simulink model "sm_DDPG_Training_Circuit_h0"  (R2022b)
settings: Solver=VariableStepAuto  StartTime=0.0  StopTime=2000  RelTol=1e-3
values from neighbouring files (symbols this model uses):
  areaFinEvap = 0.05    [pramInit.m]
  areaRoofRoom1 = roofArea/4    [pramInit.m]
  areaRoofRoom2 = roofArea/4    [pramInit.m]
  areaRoofRoom3 = roofArea/4    [pramInit.m]
  areaRoofRoom4 = roofArea/4    [pramInit.m]
  areaWallRoom1 = (lenHouse*3/5 *htHouse+widHouse*2/3*htHouse) - areaWindowRoom1    (= 95.6666666667)    [pramInit.m]
  areaWallRoom2 = (lenHouse*3/5*htHouse+widHouse/3*htHouse) - areaWindowRoom2    (= 83.3333333333)    [pramInit.m]
  areaWallRoom3 = (lenHouse*2/5*htHouse+widHouse*2/3*htHouse) - areaWindowRoom3    (= 72.6666666667)    [pramInit.m]
  areaWallRoom4 = (lenHouse*2/5*htHouse+widHouse/3*htHouse) - areaWindowRoom4    (= 59.3333333333)    [pramInit.m]
  areaWindowRoom1 = 3 * 1 *1    (= 3)    [pramInit.m]
  areaWindowRoom2 = 2 * 1 *1    (= 2)    [pramInit.m]
  areaWindowRoom3 = 2* 1 *1    (= 2)    [pramInit.m]
  areaWindowRoom4 = 2 * 1 *1    (= 2)    [pramInit.m]
  diaCond = 0.014    [pramInit.m]
  diaEvap = 0.126    [pramInit.m]
  diaGroundLoop = 0.032    [pramInit.m]
  diaOuterCond = 0.0158    [pramInit.m]
  diaOuterEvap = 0.1344    [pramInit.m]
  diaRadiatorPipe = 0.0125    [pramInit.m]
  htCondDuct = 0.3    [pramInit.m]
  htEvapDuct = 2.5    [pramInit.m]
  kTube = 400    [pramInit.m]
  leakRoofPercent = 0.1    [pramInit.m]
  leakWallPercent = 0.15    [pramInit.m]
  leakWinPercent = 0.2    [pramInit.m]
  numFinsEvap = 90    [pramInit.m]
  numTubeRowsCond = 20    [pramInit.m]
  numTubeRowsEvap = 400    [pramInit.m]
  numTubesPerRowCond = 10    [pramInit.m]
  numTubesPerRowEvap = 20    [pramInit.m]
  qGroundLoopPump = 18    [pramInit.m]
  roofDensity = 32    [pramInit.m]
  thkRoof = 0.2    [pramInit.m]
  thkWall = 0.2    [pramInit.m]
  thkWindow = 0.01    [pramInit.m]
  tInitHW = 50    [pramInit.m]
  tRoom = 23    [pramInit.m]
  Ts = 1.0    (= 1)    [code_DDPG_Training.m]    (also in code_Experimental_Setup.m)
  wallDensity = 1920    [pramInit.m]
  wCondDuct = 1.6    [pramInit.m]
  wEvapDuct = 0.96    [pramInit.m]
  windowDensity = 2700    [pramInit.m]
undefined symbols (not defined in the file or in its folder): DiscIntNeverNeededParam
libraries: fl_lib x144, nesl_utility x27, SimscapeFluids_lib x15, simulink x4, rllib x1
(part 2 of 4)

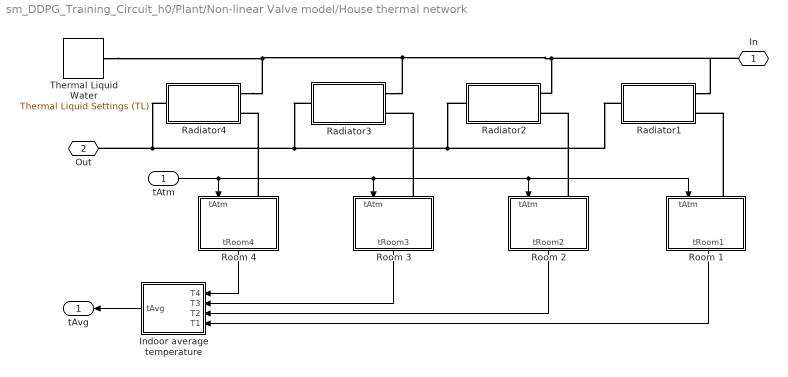
== system sm_DDPG_Training_Circuit_h0/Plant/Non-linear Valve model/House thermal network ==
  tAtm : Inport
  Indoor average temperature : Subsystem
  Radiator1 : Subsystem
      mask Display: disp('Radiator')
  Radiator2 : Subsystem
      mask Display: disp('Radiator')
  Radiator3 : Subsystem
      mask Display: disp('Radiator')
  Radiator4 : Subsystem
      mask Display: disp('Radiator')
  Room 1 : Subsystem  Tag=PublishSubsystem
      mask Display: disp('Room 1')
  Room 2 : Subsystem  Tag=PublishSubsystem
      mask Display: disp('Room 2')
  Room 3 : Subsystem  Tag=PublishSubsystem
      mask Display: disp('Room 3')
  Room 4 : Subsystem  Tag=PublishSubsystem
      mask Display: disp('Room 4')
  Thermal Liquid Water : fl_lib/Thermal Liquid/Utilities/Thermal Liquid Settings (TL)  table_dimensions=0  T_TLU=[273.1600 : 10 : 373.16]' K  p_TLU=[0.01, 0.1, 5 : 5 : 50] MPa  p_atm=0.101325 MPa  pT_region_flag=1  T_min=273.16 K  T_max=373.16 K  p_min=0.01 MPa  p_max=50 MPa  T_min_1D=273.16 K  T_max_1D=363.16 K  p_min_1D=0.05 MPa  p_max_1D=50 MPa  pT_validity_TLU=[1, 1, 1, 1, 1, 1, 1, 1, 1, 1, 1, 1; 1, 1, 1, 1, 1, 1, 1, 1, 1, 1, 1, 1; 1, 1, 1, 1, 1, 1, 1, 1, 1, 1, 1, 1; 1, 1, 1, 1, 1, 1, 1, 1, 1, 1, 1, 1; 1, 1, 1, 1, 1, 1, 1, 1, 1, 1, 1, 1; 0, 1, 1, 1, 1, 1, 1, 1, 1, 1, 1, 1; 0, 1, 1, 1, 1, 1, 1, 1, 1, 1, 1, 1; 0, 1, 1, 1, 1, 1, 1, 1, 1, 1, 1, 1; 0, 1, 1, 1, 1, 1, 1, 1, 1, 1, 1, 1; 0, 1, 1, 1, 1, 1, 1, 1, 1, 1, 1, 1; 0, 1, 1, 1, 1, 1, 1, 1, 1, 1, 1, 1]  rho_parameterization_2D=1  rho_parameterization_1D=1  rho_TLU=[999.8, 999.8, 1002.3, 1004.8, 1007.3, 1009.7, 1012.2, 1014.5, 1016.9, 1019.2, 1021.5, 1023.8; 999.7, 999.7, 1002.0, 1004.4, 1006.7, 1009.0, 1011.3, 1013.5, 1015.8, 1018.0, 1020.2, 1022.3; 998.2, 998.2, 1000.4, 1002.7, 1004.9, 1007.1, 1009.3, 1011.5, 1013.6, 1015.7, 1017.8, 1019.9; 995.6, 995.6, 997.8, 1000.0, 1002.2, 1004.3, 1006.5, 1008.6, 1010.7, 1012.7, 1014.8, 1016.8; 992.2, 992.2, 994.4, 996.5, 998.6, 1000.8, 1002.9, 1004.9, 1007.0, 1009.0, 1011.0, 1013.0; 988.0, 988.0, 990.2, 992.3, 994.4, 996.5, 998.6, 1000.7, 1002.7, 1004.7, 1006.7, 1008.7; 983.2, 983.2, 985.3, 987.5, 989.6, 991.7, 993.8, 995.8, 997.9, 999.9, 1001.9, 1003.9; 977.8, 977.8, 979.9, 982.1, 984.2, 986.3, 988.4, 990.5, 992.5, 994.6, 996.6, 998.6; 971.8, 971.8, 974.0, 976.2, 978.3, 980.5, 982.6, 984.7, 986.8, 988.8, 990.9, 992.9; 965.3, 965.3, 967.5, 969.8, 972.0, 974.2, 976.3, 978.5, 980.6, 982.7, 984.7, 986.8; 958.8, 958.8, 960.6, 962.9, 965.2, 967.4, 969.6, 971.8, 974.0, 976.1, 978.2, 980.3] kg/m^3  beta_TLU=[1.9649, 1.9654, 1.9929, 2.0213, 2.0499, 2.0787, 2.1078, 2.1372, 2.1668, 2.1966, 2.2268, 2.2572; 2.0913, 2.0918, 2.1191, 2.1471, 2.1752, 2.2036, 2.2322, 2.2610, 2.2899, 2.3191, 2.3485, 2.3781; 2.1786, 2.1791, 2.2067, 2.2350, 2.2634, 2.2919, 2.3206, 2.3494, 2.3784, 2.4075, 2.4367, 2.4661; 2.2332, 2.2337, 2.2619, 2.2908, 2.3197, 2.3487, 2.3778, 2.4070, 2.4363, 2.4657, 2.4951, 2.5246; 2.2600, 2.2605, 2.2895, 2.3191, 2.3487, 2.3784, 2.4081, 2.4378, 2.4675, 2.4973, 2.5272, 2.5571; 2.2638, 2.2638, 2.2936, 2.3240, 2.3544, 2.3848, 2.4151, 2.4455, 2.4758, 2.5062, 2.5365, 2.5669; 2.2472, 2.2472, 2.2779, 2.3092, 2.3403, 2.3715, 2.4025, 2.4336, 2.4646, 2.4955, 2.5264, 2.5573; 2.2140, 2.2140, 2.2455, 2.2776, 2.3096, 2.3415, 2.3733, 2.4050, 2.4367, 2.4683, 2.4998, 2.5313; 2.1668, 2.1668, 2.1992, 2.2321, 2.2649, 2.2976, 2.3301, 2.3626, 2.3949, 2.4272, 2.4593, 2.4914; 2.1081, 2.1081, 2.1413, 2.1750, 2.2086, 2.2421, 2.2754, 2.3085, 2.3415, 2.3744, 2.4072, 2.4399; 2.0494, 2.0494, 2.0739, 2.1084, 2.1428, 2.1770, 2.2110, 2.2449, 2.2786, 2.3121, 2.3455, 2.3788] GPa  alpha_TLU=(1e-4 * [- 0.6790, - 0.6760, - 0.4900, - 0.3070, - 0.1300, 0.0410, 0.2060, 0.3650, 0.5190, 0.6680, 0.8110, 0.9490; 0.8780, 0.8810, 0.9980, 1.1140, 1.2270, 1.3370, 1.4450, 1.5490, 1.6510, 1.7500, 1.8460, 1.9390; 2.0680, 2.0690, 2.1410, 2.2130, 2.2830, 2.3520, 2.4200, 2.4860, 2.5510, 2.6140, 2.6760, 2.7360; 3.0340, 3.0350, 3.0740, 3.1130, 3.1520, 3.1910, 3.2290, 3.2670, 3.3050, 3.3410, 3.3770, 3.4130; 3.8550, 3.8560, 3.8700, 3.8840, 3.8990, 3.9140, 3.9300, 3.9460, 3.9610, 3.9770, 3.9930, 4.0090; 4.5780, 4.5780, 4.5720, 4.5660, 4.5620, 4.5580, 4.5550, 4.5520, 4.5500, 4.5490, 4.5480, 4.5470; 5.2330, 5.2330, 5.2090, 5.1860, 5.1650, 5.1440, 5.1250, 5.1070, 5.0900, 5.0740, 5.0590, 5.0450; 5.8400, 5.8400, 5.8010, 5.7620, 5.7250, 5.6910, 5.6570, 5.6250, 5.5950, 5.5660, 5.5380, 5.5120; 6.4140, 6.4140, 6.3600, 6.3070, 6.2560, 6.2080, 6.1610, 6.1170, 6.0740, 6.0330, 5.9940, 5.9560; 6.9670, 6.9670, 6.8980, 6.8310, 6.7660, 6.7050, 6.6460, 6.5890, 6.5350, 6.4820, 6.4320, 6.3840; 7.5190, 7.5190, 7.4230, 7.3420, 7.2640, 7.1890, 7.1180, 7.0490, 6.9830, 6.9200, 6.8590, 6.8000]) 1/K  rho_TLU_2=[999.7973, 999.8431, 1002.3216, 1004.8218, 1007.293, 1009.7358, 1012.1506, 1014.5379, 1016.8979, 1019.2311, 1021.538, 1023.8188; 999.6579, 999.7009, 1002.0303, 1004.382, 1006.7084, 1009.0101, 1011.2874, 1013.5407, 1015.7703, 1017.9766, 1020.1599, 1022.3206; 998.1632, 998.2045, 1000.4375, 1002.6924, 1004.9239, 1007.1324, 1009.3183, 1011.4819, 1013.6236, 1015.7438, 1017.8428, 1019.921; 995.6057, 995.6458, 997.81864, 1000.0128, 1002.1841, 1004.3332, 1006.4603, 1008.566, 1010.6505, 1012.7144, 1014.758, 1016.7815; 992.1724, 992.2119, 994.35133, 996.5113, 998.6484, 1000.7633, 1002.8563, 1004.928, 1006.9788, 1009.009, 1011.0192, 1013.0097; 988.02, 988.0299, 990.15684, 992.3035, 994.4268, 996.5273, 998.6056, 1000.6622, 1002.6976, 1004.7123, 1006.7067, 1008.6813; 983.18, 983.1901, 985.3217, 987.4721, 989.5983, 991.7008, 993.7803, 995.8374, 997.8726, 999.8864, 1001.8795, 1003.8522; 977.75, 977.7583, 979.9094, 982.0783, 984.2216, 986.34, 988.4343, 990.505, 992.5529, 994.5786, 996.5825, 998.5654; 971.77, 971.7836, 973.96734, 976.1678, 978.3409, 980.4876, 982.6087, 984.7049, 986.7768, 988.8254, 990.8511, 992.8545; 965.26, 965.3023, 967.53107, 969.7753, 971.9901, 974.1764, 976.3354, 978.4676, 980.5741, 982.6556, 984.7129, 986.7465; 958.62, 958.6315, 960.627, 962.9267, 965.1944, 967.4314, 969.6387, 971.8173, 973.9681, 976.0921, 978.19, 980.2628] kg/m^3  rho_ref_3=998.21 kg/m^3  T_ref_3=293.16 K  p_ref_3=0.101325 MPa  beta_const_3=2.1791 GPa  alpha_const_3=2.0691e-4 1/K  rho_TLU_4=[999.84; 999.7; 998.2; 995.65; 992.21; 988.03; 983.19; 977.76; 971.78; 965.3; 958.8] kg/m^3  beta_const_4=2.1791 GPa  p_ref_4=0.101325 MPa  rho_ref_5=998.21 kg/m^3  T_ref_5=293.16 K  p_ref_5=0.101325 MPa  beta_const_5=2.1791 GPa  alpha_const_5=2.0691e-4 1/K  u_parameterization_2D=1  u_parameterization_1D=1  u_TLU=[0.0002, 0.0018, 0.0860, 0.1588, 0.2190, 0.2670, 0.3034, 0.3288, 0.3436, 0.3483, 0.3435, 0.3294; 42.0620, 42.0600, 41.9350, 41.8040, 41.6680, 41.5270, 41.3820, 41.2330, 41.0810, 40.9240, 40.7630, 40.5990; 83.9530, 83.9480, 83.6510, 83.3490, 83.0490, 82.7490, 82.4510, 82.1530, 81.8560, 81.5600, 81.2650, 80.9710; 125.7700, 125.7600, 125.3100, 124.8600, 124.4100, 123.9700, 123.5300, 123.1000, 122.6800, 122.2500, 121.8400, 121.4200; 167.5700, 167.5600, 166.9600, 166.3700, 165.7900, 165.2100, 164.6500, 164.0900, 163.5400, 163.0000, 162.4600, 161.9400; 209.3600, 209.3600, 208.6300, 207.9000, 207.1900, 206.4800, 205.7900, 205.1100, 204.4500, 203.7900, 203.1400, 202.5000; 251.1900, 251.1900, 250.3300, 249.4700, 248.6200, 247.7900, 246.9800, 246.1800, 245.3900, 244.6200, 243.8600, 243.1200; 293.0600, 293.0600, 292.0700, 291.0700, 290.1000, 289.1400, 288.2000, 287.2800, 286.3800, 285.4900, 284.6200, 283.7700; 334.9900, 334.9900, 333.8600, 332.7300, 331.6300, 330.5400, 329.4800, 328.4400, 327.4100, 326.4100, 325.4300, 324.4600; 377.0000, 377.0000, 375.7300, 374.4600, 373.2200, 372.0000, 370.8100, 369.6400, 368.5000, 367.3800, 366.2700, 365.1900; 419.0100, 419.0100, 417.6900, 416.2700, 414.8900, 413.5400, 412.2100, 410.9100, 409.6400, 408.4000, 407.1700, 405.9800] kJ/kg  cp_TLU=[4.2199, 4.2194, 4.1957, 4.1726, 4.1508, 4.1300, 4.1103, 4.0916, 4.0738, 4.0569, 4.0408, 4.0254; 4.1955, 4.1951, 4.1769, 4.1592, 4.1422, 4.1259, 4.1103, 4.0954, 4.0812, 4.0676, 4.0545, 4.0421; 4.1843, 4.1840, 4.1690, 4.1543, 4.1401, 4.1264, 4.1133, 4.1007, 4.0885, 4.0768, 4.0656, 4.0548; 4.1801, 4.1798, 4.1667, 4.1538, 4.1413, 4.1293, 4.1177, 4.1064, 4.0956, 4.0851, 4.0750, 4.0653; 4.1796, 4.1794, 4.1675, 4.1558, 4.1444, 4.1334, 4.1227, 4.1123, 4.1023, 4.0926, 4.0832, 4.0741; 4.1813, 4.1813, 4.1702, 4.1592, 4.1484, 4.1380, 4.1279, 4.1181, 4.1086, 4.0993, 4.0903, 4.0816; 4.1850, 4.1850, 4.1742, 4.1636, 4.1532, 4.1432, 4.1334, 4.1239, 4.1146, 4.1056, 4.0969, 4.0884; 4.1901, 4.1901, 4.1795, 4.1690, 4.1588, 4.1489, 4.1393, 4.1299, 4.1207, 4.1118, 4.1032, 4.0947; 4.1968, 4.1968, 4.1862, 4.1757, 4.1655, 4.1555, 4.1458, 4.1364, 4.1273, 4.1183, 4.1096, 4.1012; 4.2052, 4.2052, 4.1944, 4.1837, 4.1733, 4.1632, 4.1534, 4.1438, 4.1345, 4.1255, 4.1166, 4.1080; 4.2136, 4.2136, 4.2045, 4.1935, 4.1828, 4.1724, 4.1623, 4.1524, 4.1429, 4.1335, 4.1245, 4.1157] kJ/kg/K  u_TLU_2=[.0002, .0018, .086, .1588, .219, .267, .3034, .3288, .3436, .3483, .3435, .3294; 42.062, 42.06, 41.935, 41.804, 41.668, 41.527, 41.382, 41.233, 41.081, 40.924, 40.763, 40.599; 83.953, 83.948, 83.651, 83.349, 83.049, 82.749, 82.451, 82.153, 81.856, 81.56, 81.265, 80.971; 125.77, 125.76, 125.31, 124.86, 124.41, 123.97, 123.53, 123.1, 122.68, 122.25, 121.84, 121.42; 167.57, 167.56, 166.96, 166.37, 165.79, 165.21, 164.65, 164.09, 163.54, 163, 162.46, 161.94; 209.36, 209.36, 208.63, 207.9, 207.19, 206.48, 205.79, 205.11, 204.45, 203.79, 203.14, 202.5; 251.19, 251.19, 250.33, 249.47, 248.62, 247.79, 246.98, 246.18, 245.39, 244.62, 243.86, 243.12; 293.06, 293.06, 292.07, 291.07, 290.1, 289.14, 288.2, 287.28, 286.38, 285.49, 284.62, 283.77; 334.99, 334.99, 333.86, 332.73, 331.63, 330.54, 329.48, 328.44, 327.41, 326.41, 325.43, 324.46; 377, 377, 375.73, 374.46, 373.22, 372, 370.81, 369.64, 368.5, 367.38, 366.27, 365.19; 419.01, 419.01, 417.69, 416.27, 414.89, 413.54, 412.21, 410.91, 409.64, 408.4, 407.17, 405.98] kJ/kg  cp_TLU_3=[4.2199, 4.2194, 4.1957, 4.1726, 4.1508, 4.13, 4.1103, 4.0916, 4.0738, 4.0569, 4.0408, 4.0254; 4.1955, 4.1951, 4.1769, 4.1592, 4.1422, 4.1259, 4.1103, 4.0954, 4.0812, 4.0676, 4.0545, 4.0421; 4.1843, 4.184, 4.169, 4.1543, 4.1401, 4.1264, 4.1133, 4.1007, 4.0885, 4.0768, 4.0656, 4.0548; 4.1801, 4.1798, 4.1667, 4.1538, 4.1413, 4.1293, 4.1177, 4.1064, 4.0956, 4.0851, 4.075, 4.0653; 4.1796, 4.1794, 4.1675, 4.1558, 4.1444, 4.1334, 4.1227, 4.1123, 4.1023, 4.0926, 4.0832, 4.0741; 4.1813, 4.1813, 4.1702, 4.1592, 4.1484, 4.138, 4.1279, 4.1181, 4.1086, 4.0993, 4.0903, 4.0816; 4.185, 4.185, 4.1742, 4.1636, 4.1532, 4.1432, 4.1334, 4.1239, 4.1146, 4.1056, 4.0969, 4.0884; 4.1901, 4.1901, 4.1795, 4.169, 4.1588, 4.1489, 4.1393, 4.1299, 4.1207, 4.1118, 4.1032, 4.0947; 4.1968, 4.1968, 4.1862, 4.1757, 4.1655, 4.1555, 4.1458, 4.1364, 4.1273, 4.1183, 4.1096, 4.1012; 4.2052, 4.2052, 4.1944, 4.1837, 4.1733, 4.1632, 4.1534, 4.1438, 4.1345, 4.1255, 4.1166, 4.108; 4.2136, 4.2136, 4.2045, 4.1935, 4.1828, 4.1724, 4.1623, 4.1524, 4.1429, 4.1335, 4.1245, 4.1157] kJ/kg/K  u_TLU_4=[.0018; 42.06; 83.948; 125.76; 167.56; 209.36; 251.19; 293.06; 334.99; 377; 418.01] kJ/kg  cp_TLU_5=[4.2199; 4.1955; 4.1843; 4.1801; 4.1796; 4.1813; 4.185; 4.1901; 4.1968; 4.2052; 4.2136] kJ/kg/K  nu_TLU=[1.7917, 1.7914, 1.7763, 1.7615, 1.7473, 1.7338, 1.7208, 1.7085, 1.6967, 1.6854, 1.6747, 1.6645; 1.3061, 1.3059, 1.2986, 1.2914, 1.2845, 1.2779, 1.2716, 1.2656, 1.2598, 1.2543, 1.2491, 1.2441; 1.0032, 1.0032, 0.9995, 0.9959, 0.9924, 0.9891, 0.9859, 0.9829, 0.9801, 0.9774, 0.9748, 0.9724; 0.8006, 0.8005, 0.7987, 0.7970, 0.7953, 0.7937, 0.7922, 0.7908, 0.7894, 0.7881, 0.7870, 0.7859; 0.6577, 0.6577, 0.6570, 0.6562, 0.6555, 0.6548, 0.6543, 0.6537, 0.6532, 0.6528, 0.6523, 0.6520; 0.5530, 0.5530, 0.5529, 0.5527, 0.5526, 0.5525, 0.5524, 0.5524, 0.5524, 0.5524, 0.5524, 0.5525; 0.4739, 0.4739, 0.4741, 0.4743, 0.4745, 0.4747, 0.4750, 0.4753, 0.4755, 0.4758, 0.4762, 0.4765; 0.4127, 0.4127, 0.4131, 0.4135, 0.4139, 0.4143, 0.4148, 0.4152, 0.4157, 0.4162, 0.4167, 0.4172; 0.3643, 0.3643, 0.3648, 0.3654, 0.3659, 0.3665, 0.3670, 0.3676, 0.3682, 0.3688, 0.3694, 0.3700; 0.3254, 0.3254, 0.3261, 0.3267, 0.3273, 0.3280, 0.3286, 0.3293, 0.3299, 0.3306, 0.3312, 0.3319; 0.2866, 0.2866, 0.2945, 0.2952, 0.2959, 0.2965, 0.2972, 0.2979, 0.2986, 0.2993, 0.3000, 0.3007] mm^2/s  nu_TLU_2=[1.7917; 1.3061; 1.0032; .8006; .6577; .553; .4739; .4127; .3643; .3254; .2866] mm^2/s  k_TLU=[561.0400, 561.0900, 563.8000, 566.5600, 569.3200, 572.0800, 574.8200, 577.5400, 580.2400, 582.9200, 585.5700, 588.1800; 580.0200, 580.0700, 582.4500, 584.8800, 587.3200, 589.7500, 592.1800, 594.6100, 597.0200, 599.4200, 601.8000, 604.1600; 598.4400, 598.4800, 600.7300, 603.0300, 605.3300, 607.6400, 609.9400, 612.2400, 614.5400, 616.8200, 619.1000, 621.3600; 615.4800, 615.5200, 617.7300, 620.0000, 622.2600, 624.5400, 626.8100, 629.0700, 631.3400, 633.6000, 635.8500, 638.0900; 630.6000, 630.6400, 632.8700, 635.1500, 637.4400, 639.7200, 642.0100, 644.2900, 646.5700, 648.8400, 651.1100, 653.3600; 643.6100, 643.6100, 645.8800, 648.2100, 650.5300, 652.8600, 655.1800, 657.5100, 659.8200, 662.1400, 664.4400, 666.7400; 654.3900, 654.3900, 656.7300, 659.1200, 661.5000, 663.8900, 666.2700, 668.6500, 671.0200, 673.3800, 675.7400, 678.0900; 663.1300, 663.1300, 665.5400, 668.0000, 670.4600, 672.9100, 675.3600, 677.8000, 680.2400, 682.6700, 685.0900, 687.5000; 670.0200, 670.0200, 672.5100, 675.0500, 677.5900, 680.1200, 682.6400, 685.1600, 687.6700, 690.1700, 692.6600, 695.1400; 675.2700, 675.2700, 677.8500, 680.4800, 683.1100, 685.7300, 688.3400, 690.9400, 693.5300, 696.1100, 698.6800, 701.2400; 680.5200, 680.5200, 681.7700, 684.5000, 687.2200, 689.9400, 692.6400, 695.3400, 698.0200, 700.6900, 703.3500, 706.0000] mW/m/K  k_TLU_2=[561.04; 580.02; 598.44; 615.48; 630.6; 643.61; 654.39; 663.13; 670.02; 675.27; 680.52] mW/m/K
  In : PMIOPort  Side=Left
  Out : PMIOPort  Port=2  Side=Left
  tAvg : Outport  VectorParamsAs1DForOutWhenUnconnected=off
  wires:
  Room 1/1(tRoom1) -> Indoor average temperature/4(T1)
  Room 3/1(tRoom3) -> Indoor average temperature/2(T3)
  Room 2/1(tRoom2) -> Indoor average temperature/3(T2)
  tAtm/1 -> Room 4/1(tAtm), Room 3/1(tAtm), Room 2/1(tAtm), Room 1/1(tAtm)
  Indoor average temperature/1(tAvg) -> tAvg/1
  Room 4/1(tRoom4) -> Indoor average temperature/1(T4)
  connections:
  Radiator4/LConn1 -- Thermal Liquid Water/RConn1 -- Radiator1/LConn1 -- In/RConn1 -- Radiator2/LConn1 -- Radiator3/LConn1
  Radiator2/RConn1 -- Radiator3/RConn1 -- Radiator4/RConn1 -- Out/RConn1 -- Radiator1/RConn1
  Room 3/LConn1 -- Radiator3/LConn2
  Room 2/LConn1 -- Radiator2/LConn2
  Room 4/LConn1 -- Radiator4/LConn2
  Room 1/LConn1 -- Radiator1/LConn2

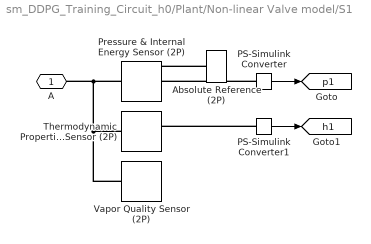
== system sm_DDPG_Training_Circuit_h0/Plant/Non-linear Valve model/S1 ==
  Absolute Reference (2P) : fl_lib/Two-Phase Fluid/Elements/Absolute Reference (2P)
  PS-Simulink Converter : nesl_utility/PS-Simulink Converter  PhysicalDomain=network_engine_domain  SubClassName=ps_output  LeftPortType=input  RightPortType=output  PseudoPeriodic=off  Frequencies=[]  VectorFormat=1-D array  Unit=MPa  AffineConversion=off
  PS-Simulink Converter1 : nesl_utility/PS-Simulink Converter  PhysicalDomain=network_engine_domain  SubClassName=ps_output  LeftPortType=input  RightPortType=output  PseudoPeriodic=off  Frequencies=[]  VectorFormat=1-D array  Unit=kJ/kg  AffineConversion=off
  Pressure & Internal Energy Sensor (2P) : fl_lib/Two-Phase Fluid/Sensors/Pressure & Internal Energy Sensor (2P)
      settings: InternalSimscapePortConfiguration="{\"Bottom\":[],\"Left\":[{\"id\":\"A\",\"label\":\"A\",\"type\":\"foundation.two_phase_fluid.two_phase_fluid\"}],\"Right\":[{\"id\":\"B\",\"label\":\"B\",\"type\":\"foundation.two_phase_fluid.two_phase_fluid\"},{\"id\":\"P\",\"label\":\"P\",\"type\":\"output\"},{\"id\":\"U\",\"label\":\"U\",\"type\":\"output\"}],\"Top\":[]}"
  Thermodynamic Properties Sensor (2P) : fl_lib/Two-Phase Fluid/Sensors/Thermodynamic Properties Sensor (2P)
      settings: InternalSimscapePortConfiguration="{\"Bottom\":[],\"Left\":[{\"id\":\"A\",\"label\":\"A\",\"type\":\"foundation.two_phase_fluid.two_phase_fluid\"}],\"Right\":[{\"id\":\"T\",\"label\":\"T\",\"type\":\"output\"},{\"id\":\"H\",\"label\":\"h\",\"type\":\"output\"},{\"id\":\"V\",\"label\":\"v\",\"type\":\"output\"},{\"id\":\"S\",\"label\":\"s\",\"type\":\"output\"}],\"Top\":[]}"
  Vapor Quality Sensor (2P) : fl_lib/Two-Phase Fluid/Sensors/Vapor Quality Sensor (2P)  vapor_fraction_spec=foundation.enum.vapor_fraction_spec.quality
      settings: InternalSimscapePortConfiguration="{\"Bottom\":[],\"Left\":[{\"id\":\"A\",\"label\":\"A\",\"type\":\"foundation.two_phase_fluid.two_phase_fluid\"}],\"Right\":[{\"id\":\"X\",\"label\":\"X\",\"type\":\"output\"}],\"Top\":[]}"
  A : PMIOPort  Side=Right
  tag scope: h1=global, p1=global
  wires:
  PS-Simulink Converter/1 -> [p1]
  PS-Simulink Converter1/1 -> [h1]
  connections:
  A/RConn1 -- Pressure & Internal Energy Sensor (2P)/LConn1 -- Vapor Quality Sensor (2P)/LConn1 -- Thermodynamic Properties Sensor (2P)/LConn1
  Absolute Reference (2P)/LConn1 -- Pressure & Internal Energy Sensor (2P)/RConn1
  PS-Simulink Converter/LConn1 -- Pressure & Internal Energy Sensor (2P)/RConn2
  PS-Simulink Converter1/LConn1 -- Thermodynamic Properties Sensor (2P)/RConn2

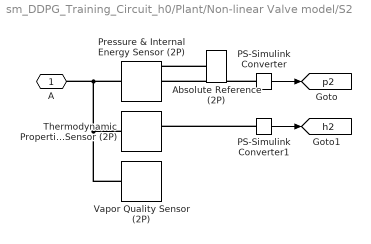
== system sm_DDPG_Training_Circuit_h0/Plant/Non-linear Valve model/S2 ==
  Absolute Reference (2P) : fl_lib/Two-Phase Fluid/Elements/Absolute Reference (2P)
  PS-Simulink Converter : nesl_utility/PS-Simulink Converter  PhysicalDomain=network_engine_domain  SubClassName=ps_output  LeftPortType=input  RightPortType=output  PseudoPeriodic=off  Frequencies=[]  VectorFormat=1-D array  Unit=MPa  AffineConversion=off
  PS-Simulink Converter1 : nesl_utility/PS-Simulink Converter  PhysicalDomain=network_engine_domain  SubClassName=ps_output  LeftPortType=input  RightPortType=output  PseudoPeriodic=off  Frequencies=[]  VectorFormat=1-D array  Unit=kJ/kg  AffineConversion=off
  Pressure & Internal Energy Sensor (2P) : fl_lib/Two-Phase Fluid/Sensors/Pressure & Internal Energy Sensor (2P)
      settings: InternalSimscapePortConfiguration="{\"Bottom\":[],\"Left\":[{\"id\":\"A\",\"label\":\"A\",\"type\":\"foundation.two_phase_fluid.two_phase_fluid\"}],\"Right\":[{\"id\":\"B\",\"label\":\"B\",\"type\":\"foundation.two_phase_fluid.two_phase_fluid\"},{\"id\":\"P\",\"label\":\"P\",\"type\":\"output\"},{\"id\":\"U\",\"label\":\"U\",\"type\":\"output\"}],\"Top\":[]}"
  Thermodynamic Properties Sensor (2P) : fl_lib/Two-Phase Fluid/Sensors/Thermodynamic Properties Sensor (2P)
      settings: InternalSimscapePortConfiguration="{\"Bottom\":[],\"Left\":[{\"id\":\"A\",\"label\":\"A\",\"type\":\"foundation.two_phase_fluid.two_phase_fluid\"}],\"Right\":[{\"id\":\"T\",\"label\":\"T\",\"type\":\"output\"},{\"id\":\"H\",\"label\":\"h\",\"type\":\"output\"},{\"id\":\"V\",\"label\":\"v\",\"type\":\"output\"},{\"id\":\"S\",\"label\":\"s\",\"type\":\"output\"}],\"Top\":[]}"
  Vapor Quality Sensor (2P) : fl_lib/Two-Phase Fluid/Sensors/Vapor Quality Sensor (2P)  vapor_fraction_spec=foundation.enum.vapor_fraction_spec.quality
      settings: InternalSimscapePortConfiguration="{\"Bottom\":[],\"Left\":[{\"id\":\"A\",\"label\":\"A\",\"type\":\"foundation.two_phase_fluid.two_phase_fluid\"}],\"Right\":[{\"id\":\"X\",\"label\":\"X\",\"type\":\"output\"}],\"Top\":[]}"
  A : PMIOPort  Side=Left
  tag scope: h2=global, p2=global
  wires:
  PS-Simulink Converter/1 -> [p2]
  PS-Simulink Converter1/1 -> [h2]
  connections:
  Absolute Reference (2P)/LConn1 -- Pressure & Internal Energy Sensor (2P)/RConn1
  Thermodynamic Properties Sensor (2P)/LConn1 -- Vapor Quality Sensor (2P)/LConn1 -- Pressure & Internal Energy Sensor (2P)/LConn1 -- A/RConn1
  PS-Simulink Converter1/LConn1 -- Thermodynamic Properties Sensor (2P)/RConn2
  PS-Simulink Converter/LConn1 -- Pressure & Internal Energy Sensor (2P)/RConn2

== system sm_DDPG_Training_Circuit_h0/Plant/Non-linear Valve model/S3 ==
  Absolute Reference (2P) : fl_lib/Two-Phase Fluid/Elements/Absolute Reference (2P)
  PS-Simulink Converter : nesl_utility/PS-Simulink Converter  PhysicalDomain=network_engine_domain  SubClassName=ps_output  LeftPortType=input  RightPortType=output  PseudoPeriodic=off  Frequencies=[]  VectorFormat=1-D array  Unit=MPa  AffineConversion=off
  PS-Simulink Converter1 : nesl_utility/PS-Simulink Converter  PhysicalDomain=network_engine_domain  SubClassName=ps_output  LeftPortType=input  RightPortType=output  PseudoPeriodic=off  Frequencies=[]  VectorFormat=1-D array  Unit=kJ/kg  AffineConversion=off
  Pressure & Internal Energy Sensor (2P) : fl_lib/Two-Phase Fluid/Sensors/Pressure & Internal Energy Sensor (2P)
      settings: InternalSimscapePortConfiguration="{\"Bottom\":[],\"Left\":[{\"id\":\"A\",\"label\":\"A\",\"type\":\"foundation.two_phase_fluid.two_phase_fluid\"}],\"Right\":[{\"id\":\"B\",\"label\":\"B\",\"type\":\"foundation.two_phase_fluid.two_phase_fluid\"},{\"id\":\"P\",\"label\":\"P\",\"type\":\"output\"},{\"id\":\"U\",\"label\":\"U\",\"type\":\"output\"}],\"Top\":[]}"
  Thermodynamic Properties Sensor (2P) : fl_lib/Two-Phase Fluid/Sensors/Thermodynamic Properties Sensor (2P)
      settings: InternalSimscapePortConfiguration="{\"Bottom\":[],\"Left\":[{\"id\":\"A\",\"label\":\"A\",\"type\":\"foundation.two_phase_fluid.two_phase_fluid\"}],\"Right\":[{\"id\":\"T\",\"label\":\"T\",\"type\":\"output\"},{\"id\":\"H\",\"label\":\"h\",\"type\":\"output\"},{\"id\":\"V\",\"label\":\"v\",\"type\":\"output\"},{\"id\":\"S\",\"label\":\"s\",\"type\":\"output\"}],\"Top\":[]}"
  Vapor Quality Sensor (2P) : fl_lib/Two-Phase Fluid/Sensors/Vapor Quality Sensor (2P)  vapor_fraction_spec=foundation.enum.vapor_fraction_spec.quality
      settings: InternalSimscapePortConfiguration="{\"Bottom\":[],\"Left\":[{\"id\":\"A\",\"label\":\"A\",\"type\":\"foundation.two_phase_fluid.two_phase_fluid\"}],\"Right\":[{\"id\":\"X\",\"label\":\"X\",\"type\":\"output\"}],\"Top\":[]}"
  A : PMIOPort  Side=Left
  tag scope: h3=global, p3=global
  wires:
  PS-Simulink Converter/1 -> [p3]
  PS-Simulink Converter1/1 -> [h3]
  connections:
  A/RConn1 -- Pressure & Internal Energy Sensor (2P)/LConn1 -- Vapor Quality Sensor (2P)/LConn1 -- Thermodynamic Properties Sensor (2P)/LConn1
  Absolute Reference (2P)/LConn1 -- Pressure & Internal Energy Sensor (2P)/RConn1
  PS-Simulink Converter/LConn1 -- Pressure & Internal Energy Sensor (2P)/RConn2
  PS-Simulink Converter1/LConn1 -- Thermodynamic Properties Sensor (2P)/RConn2

== system sm_DDPG_Training_Circuit_h0/Plant/Non-linear Valve model/S4 ==
  Absolute Reference (2P) : fl_lib/Two-Phase Fluid/Elements/Absolute Reference (2P)
  PS-Simulink Converter : nesl_utility/PS-Simulink Converter  PhysicalDomain=network_engine_domain  SubClassName=ps_output  LeftPortType=input  RightPortType=output  PseudoPeriodic=off  Frequencies=[]  VectorFormat=1-D array  Unit=MPa  AffineConversion=off
  PS-Simulink Converter1 : nesl_utility/PS-Simulink Converter  PhysicalDomain=network_engine_domain  SubClassName=ps_output  LeftPortType=input  RightPortType=output  PseudoPeriodic=off  Frequencies=[]  VectorFormat=1-D array  Unit=kJ/kg  AffineConversion=off
  Pressure & Internal Energy Sensor (2P) : fl_lib/Two-Phase Fluid/Sensors/Pressure & Internal Energy Sensor (2P)
      settings: InternalSimscapePortConfiguration="{\"Bottom\":[],\"Left\":[{\"id\":\"A\",\"label\":\"A\",\"type\":\"foundation.two_phase_fluid.two_phase_fluid\"}],\"Right\":[{\"id\":\"B\",\"label\":\"B\",\"type\":\"foundation.two_phase_fluid.two_phase_fluid\"},{\"id\":\"P\",\"label\":\"P\",\"type\":\"output\"},{\"id\":\"U\",\"label\":\"U\",\"type\":\"output\"}],\"Top\":[]}"
  Thermodynamic Properties Sensor (2P) : fl_lib/Two-Phase Fluid/Sensors/Thermodynamic Properties Sensor (2P)
      settings: InternalSimscapePortConfiguration="{\"Bottom\":[],\"Left\":[{\"id\":\"A\",\"label\":\"A\",\"type\":\"foundation.two_phase_fluid.two_phase_fluid\"}],\"Right\":[{\"id\":\"T\",\"label\":\"T\",\"type\":\"output\"},{\"id\":\"H\",\"label\":\"h\",\"type\":\"output\"},{\"id\":\"V\",\"label\":\"v\",\"type\":\"output\"},{\"id\":\"S\",\"label\":\"s\",\"type\":\"output\"}],\"Top\":[]}"
  Vapor Quality Sensor (2P) : fl_lib/Two-Phase Fluid/Sensors/Vapor Quality Sensor (2P)  vapor_fraction_spec=foundation.enum.vapor_fraction_spec.quality
      settings: InternalSimscapePortConfiguration="{\"Bottom\":[],\"Left\":[{\"id\":\"A\",\"label\":\"A\",\"type\":\"foundation.two_phase_fluid.two_phase_fluid\"}],\"Right\":[{\"id\":\"X\",\"label\":\"X\",\"type\":\"output\"}],\"Top\":[]}"
  A : PMIOPort  Side=Left
  tag scope: h4=global, p4=global
  wires:
  PS-Simulink Converter/1 -> [p4]
  PS-Simulink Converter1/1 -> [h4]
  connections:
  Absolute Reference (2P)/LConn1 -- Pressure & Internal Energy Sensor (2P)/RConn1
  Thermodynamic Properties Sensor (2P)/LConn1 -- Vapor Quality Sensor (2P)/LConn1 -- Pressure & Internal Energy Sensor (2P)/LConn1 -- A/RConn1
  PS-Simulink Converter1/LConn1 -- Thermodynamic Properties Sensor (2P)/RConn2
  PS-Simulink Converter/LConn1 -- Pressure & Internal Energy Sensor (2P)/RConn2

== system sm_DDPG_Training_Circuit_h0/Plant/Non-linear Valve model/House thermal network/Indoor average temperature ==
  T4 : Inport
  T3 : Inport  Port=2
  T2 : Inport  Port=3
  T1 : Inport  Port=4
  Gain : Gain  Gain=1/4
  Sum of Elements : Sum  Inputs=++++
  tAvg : Outport  VectorParamsAs1DForOutWhenUnconnected=off
  wires:
  T2/1 -> Sum of Elements/3
  Sum of Elements/1 -> Gain/1
  T1/1 -> Sum of Elements/4
  T4/1 -> Sum of Elements/1
  Gain/1 -> tAvg/1
  T3/1 -> Sum of Elements/2

== system sm_DDPG_Training_Circuit_h0/Plant/Non-linear Valve model/House thermal network/Radiator1 ==
  Convective Heat Transfer : fl_lib/Thermal/Thermal Elements/Convective Heat Transfer  thermal_type=foundation.enum.constant_variable.constant  area=areaRadiator1 m^2  heat_tr_coeff=hRadiator1 W/(m^2*K)  min_heat_tr_coeff=1e-3 W/(K*m^2)  T_specify=off  T_priority=None  T=0 K  T_nominal_specify=off  T_nominal_unit=K  T_nominal_value=1  Q_specify=off  Q_priority=None  Q=0 J/s  Q_nominal_specify=off  Q_nominal_unit=W  Q_nominal_value=1
  Pipe (TL) : SimscapeFluids_lib/Thermal Liquid/Pipes & Fittings/Pipe (TL)  dynamic_compressibility=simscape.enum.onoff.on  inertia=simscape.enum.onoff.off  num_segments=1  pipe_length=lenRadiatorPipe m  area=pi*0.25*(diaRadiatorPipe)^2 m^2  wall_spec=fluids.thermal_liquid.pipes_fittings.enum.wall_spec.rigid  Dh=0.1128 m  wall_compliance=1.2e-6 m/MPa  wall_time_constant=0.01 s  elevation_spec=foundation.enum.constant_variable.constant  elevation_gain=0 m  g=9.81 m/s^2  pressure_loss_spec=fluids.thermal_liquid.pipes_fittings.enum.PressureLossSpec.Haaland  local_pressure_loss_spec=fluids.thermal_liquid.pipes_fittings.enum.LocalLossSpec.AggregateLength  length_add=1 m  loss_coefficient=0.1  roughness=1.5e-5 m  Re_friction_TLU=[ 400 1000 1.5e+3 3e+3 4e+3 6e+3 1e+4 2e+4 4e+4 6e+4 1e+5 1e+8 ]  friction_factor_TLU=[ 0.264 0.112 0.07099999999999999 0.0417 0.0387 0.0268 0.025 0.0232 0.0226 0.022 0.0214 0.0214 ]  shape_factor=64  Re_lam=2e+3  Re_tur=4e+3  mdot_nominal=[ 0.1 1 ] kg/s  p_diff_nominal=[ 0.001 0.01 ] MPa  mdot_threshold=1e-6 kg/s  heat_transfer_spec=fluids.thermal_liquid.pipes_fittings.enum.HeatTransferSpec.Gnielinski  mdot_nominal_heat=[ 0.1 1 ] kg/s  T_in_nominal=[ 293.15 293.15 ] K  T_out_nominal=[ 300 300 ] K  p_in_nominal_heat=[ 0.101325 0.101325 ] MPa  T_wall_nominal=[ 303.15 303.15 ] K  a_coeff=0.023  b_Re_power=0.8  c_Pr_power=0.4  Nu_lam=3.66  Re_Colburn_TLU=[ 100 150 1000 ]  Colburn_factor_TLU=[ 0.019 0.013 0.002 ]  Re_Nu_TLU=[ 100 150 1000 ]  Pr_Nu_TLU=[ 1 10 ]  Nu_TLU=[ 3.72 4.21; 3.75 4.44; 4.21 7.15 ]  T0_vec=tRoom degC  p0_vec=pInitHW MPa  mdot0=0.1 kg/s
  Radiator thermal mass : fl_lib/Thermal/Thermal Elements/Thermal Mass  mass=46.7 kg  sp_heat=447 J/(K*kg)  num_ports=foundation.enum.numPorts2.one  T_specify=on  T_priority=Low  T=tRoom degC  T_nominal_specify=off  T_nominal_unit=K  T_nominal_value=1  Q_specify=off  Q_priority=High  Q=0 J/s  Q_nominal_specify=off  Q_nominal_unit=W  Q_nominal_value=1
  Inlet : PMIOPort  Side=Left
  Outlet : PMIOPort  Port=2  Side=Right
  Air : PMIOPort  Port=3  Side=Left
  connections:
  Convective Heat Transfer/RConn1 -- Air/RConn1
  Pipe (TL)/RConn1 -- Outlet/RConn1
  Pipe (TL)/LConn1 -- Inlet/RConn1
  Convective Heat Transfer/LConn1 -- Radiator thermal mass/LConn1 -- Pipe (TL)/LConn2

== system sm_DDPG_Training_Circuit_h0/Plant/Non-linear Valve model/House thermal network/Radiator2 ==
  Convective Heat Transfer : fl_lib/Thermal/Thermal Elements/Convective Heat Transfer  thermal_type=foundation.enum.constant_variable.constant  area=areaRadiator2 m^2  heat_tr_coeff=hRadiator2 W/(m^2*K)  min_heat_tr_coeff=1e-3 W/(K*m^2)  T_specify=off  T_priority=None  T=0 K  T_nominal_specify=off  T_nominal_unit=K  T_nominal_value=1  Q_specify=off  Q_priority=None  Q=0 J/s  Q_nominal_specify=off  Q_nominal_unit=W  Q_nominal_value=1
  Pipe (TL) : SimscapeFluids_lib/Thermal Liquid/Pipes & Fittings/Pipe (TL)  dynamic_compressibility=simscape.enum.onoff.on  inertia=simscape.enum.onoff.off  num_segments=1  pipe_length=lenRadiatorPipe m  area=pi*0.25*(diaRadiatorPipe)^2 m^2  wall_spec=fluids.thermal_liquid.pipes_fittings.enum.wall_spec.rigid  Dh=0.1128 m  wall_compliance=1.2e-6 m/MPa  wall_time_constant=0.01 s  elevation_spec=foundation.enum.constant_variable.constant  elevation_gain=0 m  g=9.81 m/s^2  pressure_loss_spec=fluids.thermal_liquid.pipes_fittings.enum.PressureLossSpec.Haaland  local_pressure_loss_spec=fluids.thermal_liquid.pipes_fittings.enum.LocalLossSpec.AggregateLength  length_add=1 m  loss_coefficient=0.1  roughness=1.5e-5 m  Re_friction_TLU=[ 400 1000 1.5e+3 3e+3 4e+3 6e+3 1e+4 2e+4 4e+4 6e+4 1e+5 1e+8 ]  friction_factor_TLU=[ 0.264 0.112 0.07099999999999999 0.0417 0.0387 0.0268 0.025 0.0232 0.0226 0.022 0.0214 0.0214 ]  shape_factor=64  Re_lam=2e+3  Re_tur=4e+3  mdot_nominal=[ 0.1 1 ] kg/s  p_diff_nominal=[ 0.001 0.01 ] MPa  mdot_threshold=1e-6 kg/s  heat_transfer_spec=fluids.thermal_liquid.pipes_fittings.enum.HeatTransferSpec.Gnielinski  mdot_nominal_heat=[ 0.1 1 ] kg/s  T_in_nominal=[ 293.15 293.15 ] K  T_out_nominal=[ 300 300 ] K  p_in_nominal_heat=[ 0.101325 0.101325 ] MPa  T_wall_nominal=[ 303.15 303.15 ] K  a_coeff=0.023  b_Re_power=0.8  c_Pr_power=0.4  Nu_lam=3.66  Re_Colburn_TLU=[ 100 150 1000 ]  Colburn_factor_TLU=[ 0.019 0.013 0.002 ]  Re_Nu_TLU=[ 100 150 1000 ]  Pr_Nu_TLU=[ 1 10 ]  Nu_TLU=[ 3.72 4.21; 3.75 4.44; 4.21 7.15 ]  T0_vec=tRoom degC  p0_vec=pInitHW MPa  mdot0=0.1 kg/s
  Radiator thermal mass : fl_lib/Thermal/Thermal Elements/Thermal Mass  mass=46.7 kg  sp_heat=447 J/(K*kg)  num_ports=foundation.enum.numPorts2.one  T_specify=on  T_priority=Low  T=tRoom degC  T_nominal_specify=off  T_nominal_unit=K  T_nominal_value=1  Q_specify=off  Q_priority=High  Q=0 J/s  Q_nominal_specify=off  Q_nominal_unit=W  Q_nominal_value=1
  Inlet : PMIOPort  Side=Left
  Outlet : PMIOPort  Port=2  Side=Right
  Air : PMIOPort  Port=3  Side=Left
  connections:
  Radiator thermal mass/LConn1 -- Pipe (TL)/LConn2 -- Convective Heat Transfer/LConn1
  Pipe (TL)/LConn1 -- Inlet/RConn1
  Pipe (TL)/RConn1 -- Outlet/RConn1
  Convective Heat Transfer/RConn1 -- Air/RConn1

== system sm_DDPG_Training_Circuit_h0/Plant/Non-linear Valve model/House thermal network/Radiator3 ==
  Convective Heat Transfer : fl_lib/Thermal/Thermal Elements/Convective Heat Transfer  thermal_type=foundation.enum.constant_variable.constant  area=areaRadiator3 m^2  heat_tr_coeff=hRadiator3 W/(m^2*K)  min_heat_tr_coeff=1e-3 W/(K*m^2)  T_specify=off  T_priority=None  T=0 K  T_nominal_specify=off  T_nominal_unit=K  T_nominal_value=1  Q_specify=off  Q_priority=None  Q=0 J/s  Q_nominal_specify=off  Q_nominal_unit=W  Q_nominal_value=1
  Pipe (TL) : SimscapeFluids_lib/Thermal Liquid/Pipes & Fittings/Pipe (TL)  dynamic_compressibility=simscape.enum.onoff.on  inertia=simscape.enum.onoff.off  num_segments=1  pipe_length=lenRadiatorPipe m  area=pi*0.25*(diaRadiatorPipe)^2 m^2  wall_spec=fluids.thermal_liquid.pipes_fittings.enum.wall_spec.rigid  Dh=0.1128 m  wall_compliance=1.2e-6 m/MPa  wall_time_constant=0.01 s  elevation_spec=foundation.enum.constant_variable.constant  elevation_gain=0 m  g=9.81 m/s^2  pressure_loss_spec=fluids.thermal_liquid.pipes_fittings.enum.PressureLossSpec.Haaland  local_pressure_loss_spec=fluids.thermal_liquid.pipes_fittings.enum.LocalLossSpec.AggregateLength  length_add=1 m  loss_coefficient=0.1  roughness=1.5e-5 m  Re_friction_TLU=[ 400 1000 1.5e+3 3e+3 4e+3 6e+3 1e+4 2e+4 4e+4 6e+4 1e+5 1e+8 ]  friction_factor_TLU=[ 0.264 0.112 0.07099999999999999 0.0417 0.0387 0.0268 0.025 0.0232 0.0226 0.022 0.0214 0.0214 ]  shape_factor=64  Re_lam=2e+3  Re_tur=4e+3  mdot_nominal=[ 0.1 1 ] kg/s  p_diff_nominal=[ 0.001 0.01 ] MPa  mdot_threshold=1e-6 kg/s  heat_transfer_spec=fluids.thermal_liquid.pipes_fittings.enum.HeatTransferSpec.Gnielinski  mdot_nominal_heat=[ 0.1 1 ] kg/s  T_in_nominal=[ 293.15 293.15 ] K  T_out_nominal=[ 300 300 ] K  p_in_nominal_heat=[ 0.101325 0.101325 ] MPa  T_wall_nominal=[ 303.15 303.15 ] K  a_coeff=0.023  b_Re_power=0.8  c_Pr_power=0.4  Nu_lam=3.66  Re_Colburn_TLU=[ 100 150 1000 ]  Colburn_factor_TLU=[ 0.019 0.013 0.002 ]  Re_Nu_TLU=[ 100 150 1000 ]  Pr_Nu_TLU=[ 1 10 ]  Nu_TLU=[ 3.72 4.21; 3.75 4.44; 4.21 7.15 ]  T0_vec=tRoom degC  p0_vec=pInitHW MPa  mdot0=0.1 kg/s
  Radiator thermal mass : fl_lib/Thermal/Thermal Elements/Thermal Mass  mass=46.7 kg  sp_heat=447 J/(K*kg)  num_ports=foundation.enum.numPorts2.one  T_specify=on  T_priority=Low  T=tRoom degC  T_nominal_specify=off  T_nominal_unit=K  T_nominal_value=1  Q_specify=off  Q_priority=High  Q=0 J/s  Q_nominal_specify=off  Q_nominal_unit=W  Q_nominal_value=1
  Inlet : PMIOPort  Side=Left
  Outlet : PMIOPort  Port=2  Side=Right
  Air : PMIOPort  Port=3  Side=Left
  connections:
  Convective Heat Transfer/RConn1 -- Air/RConn1
  Pipe (TL)/RConn1 -- Outlet/RConn1
  Pipe (TL)/LConn1 -- Inlet/RConn1
  Convective Heat Transfer/LConn1 -- Pipe (TL)/LConn2 -- Radiator thermal mass/LConn1

== system sm_DDPG_Training_Circuit_h0/Plant/Non-linear Valve model/House thermal network/Radiator4 ==
  Convective Heat Transfer : fl_lib/Thermal/Thermal Elements/Convective Heat Transfer  thermal_type=foundation.enum.constant_variable.constant  area=areaRadiator4 m^2  heat_tr_coeff=hRadiator4 W/(m^2*K)  min_heat_tr_coeff=1e-3 W/(K*m^2)  T_specify=off  T_priority=None  T=0 K  T_nominal_specify=off  T_nominal_unit=K  T_nominal_value=1  Q_specify=off  Q_priority=None  Q=0 J/s  Q_nominal_specify=off  Q_nominal_unit=W  Q_nominal_value=1
  Pipe (TL) : SimscapeFluids_lib/Thermal Liquid/Pipes & Fittings/Pipe (TL)  dynamic_compressibility=simscape.enum.onoff.on  inertia=simscape.enum.onoff.off  num_segments=1  pipe_length=lenRadiatorPipe m  area=pi*0.25*(diaRadiatorPipe)^2 m^2  wall_spec=fluids.thermal_liquid.pipes_fittings.enum.wall_spec.rigid  Dh=0.1128 m  wall_compliance=1.2e-6 m/MPa  wall_time_constant=0.01 s  elevation_spec=foundation.enum.constant_variable.constant  elevation_gain=0 m  g=9.81 m/s^2  pressure_loss_spec=fluids.thermal_liquid.pipes_fittings.enum.PressureLossSpec.Haaland  local_pressure_loss_spec=fluids.thermal_liquid.pipes_fittings.enum.LocalLossSpec.AggregateLength  length_add=1 m  loss_coefficient=0.1  roughness=1.5e-5 m  Re_friction_TLU=[ 400 1000 1.5e+3 3e+3 4e+3 6e+3 1e+4 2e+4 4e+4 6e+4 1e+5 1e+8 ]  friction_factor_TLU=[ 0.264 0.112 0.07099999999999999 0.0417 0.0387 0.0268 0.025 0.0232 0.0226 0.022 0.0214 0.0214 ]  shape_factor=64  Re_lam=2e+3  Re_tur=4e+3  mdot_nominal=[ 0.1 1 ] kg/s  p_diff_nominal=[ 0.001 0.01 ] MPa  mdot_threshold=1e-6 kg/s  heat_transfer_spec=fluids.thermal_liquid.pipes_fittings.enum.HeatTransferSpec.Gnielinski  mdot_nominal_heat=[ 0.1 1 ] kg/s  T_in_nominal=[ 293.15 293.15 ] K  T_out_nominal=[ 300 300 ] K  p_in_nominal_heat=[ 0.101325 0.101325 ] MPa  T_wall_nominal=[ 303.15 303.15 ] K  a_coeff=0.023  b_Re_power=0.8  c_Pr_power=0.4  Nu_lam=3.66  Re_Colburn_TLU=[ 100 150 1000 ]  Colburn_factor_TLU=[ 0.019 0.013 0.002 ]  Re_Nu_TLU=[ 100 150 1000 ]  Pr_Nu_TLU=[ 1 10 ]  Nu_TLU=[ 3.72 4.21; 3.75 4.44; 4.21 7.15 ]  T0_vec=tRoom degC  p0_vec=pInitHW MPa  mdot0=0.1 kg/s
  Radiator thermal mass : fl_lib/Thermal/Thermal Elements/Thermal Mass  mass=46.7 kg  sp_heat=447 J/(K*kg)  num_ports=foundation.enum.numPorts2.one  T_specify=on  T_priority=Low  T=tRoom degC  T_nominal_specify=off  T_nominal_unit=K  T_nominal_value=1  Q_specify=off  Q_priority=High  Q=0 J/s  Q_nominal_specify=off  Q_nominal_unit=W  Q_nominal_value=1
  Inlet : PMIOPort  Side=Left
  Outlet : PMIOPort  Port=2  Side=Right
  Air : PMIOPort  Port=3  Side=Left
  connections:
  Radiator thermal mass/LConn1 -- Pipe (TL)/LConn2 -- Convective Heat Transfer/LConn1
  Pipe (TL)/LConn1 -- Inlet/RConn1
  Pipe (TL)/RConn1 -- Outlet/RConn1
  Convective Heat Transfer/RConn1 -- Air/RConn1
